simulink subsystem "HEVP0SSC"  (R2024a)
settings: Solver=VariableStepAuto  StartTime=0.0  StopTime=10.0  RelTol=1e-3
undefined symbols (not defined in the file): PlntEngInertia
libraries: fl_lib x2, sdl_lib x1
settings Model: ModifiedByFormat=The MathWorks, Inc.  Creator=The MathWorks, Inc.  LastModifiedBy=The MathWorks, Inc.
settings OptimizationCC: ReuseModelBlockBuffer=off
settings RTWCC: GPUComputeCapability=3.5

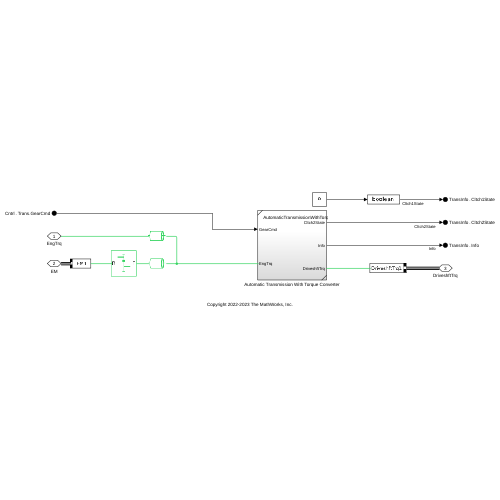
[thumbnail: Simulink's stored preview of the top-level diagram]
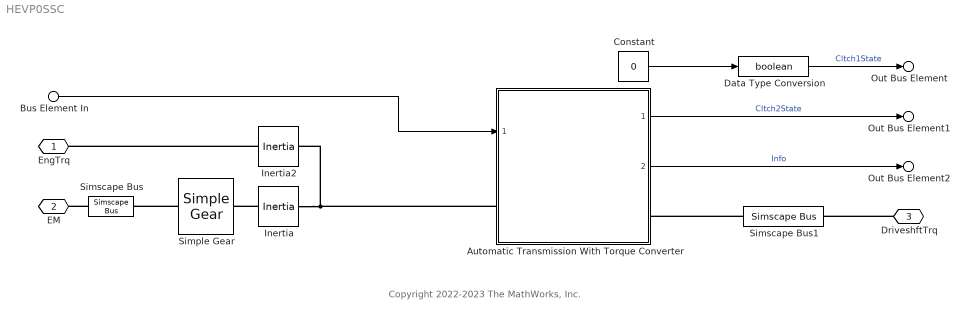
== system HEVP0SSC ==
  note: Copyright 2022-2023 The MathWorks, Inc.
  Bus Element In : Inport  PortName=Cntrl  Element=Trans.GearCmd
  Automatic Transmission With Torque Converter : Subsystem  ReferencedSubsystem=AutomaticTransmissionWithTorqueConverterSSC
  Constant : Constant  Value=0  SampleTime=-1
  Data Type Conversion : DataTypeConversion  OutDataTypeStr=boolean  SaturateOnIntegerOverflow=off  RndMeth=Floor
  Inertia : fl_lib/Mechanical/Rotational Elements/Inertia  inertia=PlntEM1Inertia kg*m^2  num_ports=foundation.enum.numPorts2.two  w_specify=off  w_priority=High  w=0 rad/s  w_nominal_specify=off  w_nominal_value=1  w_nominal_unit=rad/s  t_specify=off  t_priority=None  t=0 N*m  t_nominal_specify=off  t_nominal_value=1  t_nominal_unit=N*m
      settings: InternalSimscapePortConfiguration="{\"Bottom\":[],\"Left\":[{\"id\":\"I\",\"label\":\"\",\"type\":\"foundation.mechanical.rotational.rotational\"}],\"Right\":[{\"id\":\"J\",\"label\":\"\",\"type\":\"foundation.mechanical.rotational.rotational\"}],\"Top\":[]}"
  Inertia2 : fl_lib/Mechanical/Rotational Elements/Inertia  inertia=PlntEngInertia/2 kg*m^2  num_ports=foundation.enum.numPorts2.two  w_specify=off  w_priority=High  w=0 rad/s  w_nominal_specify=off  w_nominal_value=1  w_nominal_unit=rad/s  t_specify=off  t_priority=None  t=0 N*m  t_nominal_specify=off  t_nominal_value=1  t_nominal_unit=N*m
      settings: InternalSimscapePortConfiguration="{\"Bottom\":[],\"Left\":[{\"id\":\"I\",\"label\":\"\",\"type\":\"foundation.mechanical.rotational.rotational\"}],\"Right\":[{\"id\":\"J\",\"label\":\"\",\"type\":\"foundation.mechanical.rotational.rotational\"}],\"Top\":[]}"
  Simple Gear : sdl_lib/Gears/Simple Gear  ratio=PlntDiffrntlP0Ratio  rotation_direction=sdl.enum.shaftOutputDirection.same  enable_faults=simscape.enum.onoff.off  efficiency_fault=0.05  fault_angles=pi / 12 rad  friction_model=sdl.enum.gear_efficiencies_load.constant  T_noload=0.1 N*m  T_nom=5 N*m  efficiency_nom=0.8  efficiency=PlntP0GearEff  temperature_TLU=[280, 300, 320] K  load_TLU=[1, 5, 10] N*m  efficiency_TLU=[.95, .9, .85]  efficiency_TLU2=[.85, .8, .75; .95, .9, .85; .85, .8, .7]  w_thr=0.01 rad/s  pwr_thr=PlntP0GearPwrThresh W  enable_backlash=false  hardstop_model=simscape.enum.hardstop.smooth  backlash_distance=1e-3 mm  r_base=0.1 m  transition=1e-4 mm  backlash_stiffness=1e7 N/m  backlash_damping=1e6 N*s/m  coeff_rest=0  v_tol=0.001 m/s  f_tol=0 N  mu_visc=PlntP0GearViscFric N*m*s/rad  thermal_mass=50 J/K  temperature_specify=off  temperature_priority=High  temperature=300 K  temperature_nominal_specify=off  temperature_nominal_value=1  temperature_nominal_unit=K  x_backlash_specify=off  x_backlash_priority=None  x_backlash=0 mm  x_backlash_nominal_specify=off  x_backlash_nominal_value=1  x_backlash_nominal_unit=mm  f_hardstop_specify=off  f_hardstop_priority=None  f_hardstop=0 N  f_hardstop_nominal_specify=off  f_hardstop_nominal_value=1  f_hardstop_nominal_unit=N  v_backlash_specify=off  v_backlash_priority=None  v_backlash=0 m/s  v_backlash_nominal_specify=off  v_backlash_nominal_value=1  v_backlash_nominal_unit=m/s
  Simscape Bus : SimscapeBus  HierarchyStrings=EM1
  Simscape Bus1 : SimscapeBus  HierarchyStrings=DriveshftTrq1
  EngTrq : PMIOPort  Side=Left
  EM : PMIOPort  Port=2  Side=Left
  DriveshftTrq : PMIOPort  Port=3  Side=Right
  Out Bus Element : Outport  PortName=TransInfo  Element=Cltch1State
  Out Bus Element1 : Outport  PortName=TransInfo  Element=Cltch2State
  Out Bus Element2 : Outport  PortName=TransInfo  Element=Info
  wires:
  Bus Element In/1 -> Automatic Transmission With Torque Converter/1
  Automatic Transmission With Torque Converter/1 -> Out Bus Element1/1  "Cltch2State"
  Constant/1 -> Data Type Conversion/1
  Automatic Transmission With Torque Converter/2 -> Out Bus Element2/1  "Info"
  Data Type Conversion/1 -> Out Bus Element/1  "Cltch1State"
  connections:
  Automatic Transmission With Torque Converter/LConn1 -- Inertia2/LConn1 -- Inertia/LConn1
  Simple Gear/LConn1 -- Simscape Bus/LConn1
  Simscape Bus/RConn1 -- EM/RConn1
  DriveshftTrq/RConn1 -- Simscape Bus1/RConn1
  Simscape Bus1/LConn1 -- Automatic Transmission With Torque Converter/RConn1
  Inertia/RConn1 -- Simple Gear/RConn1
  Inertia2/RConn1 -- EngTrq/RConn1
